simulink model "RADTRANS003"  (R2020b)
settings: Solver=VariableStepAuto  StartTime=0.0  StopTime=10.0  RelTol=1e-3
undefined symbols (not defined in the file): L_street, Line_110_C, Line_110_L, Line_110_R, Line_220_C, Line_220_L, Line_220_R, Line_35_C, Line_35_L, Line_35_R, Line_6_L, Line_6_R, P_nom_dyn, Q_nom_dyn, R_street, Sys_f_Hz, Sys_V_net_kV, Tr_110_35_L_pu, Tr_110_35_R_pu, Tr_110_35_Sn_VA, Tr_110_35_V_HV_kV, Tr_110_35_V_LV_kV, Tr_110_6_L_pu, Tr_110_6_R_pu, Tr_110_6_Sn_VA, Tr_110_6_V_HV_kV, Tr_110_6_V_LV_kV, Tr_220_110_L_pu, Tr_220_110_R_pu, Tr_220_110_Sn_VA, Tr_220_110_V_HV_kV, Tr_220_110_V_LV_kV, Tr_35_04_L_pu, Tr_35_04_R_pu, Tr_35_04_Sn_VA, Tr_35_04_V_HV_kV, Tr_35_04_V_LV_kV, Tr_6_04_L_pu, Tr_6_04_R_pu, Tr_6_04_Sn_VA, Tr_6_04_V_HV_kV, Tr_6_04_V_LV_kV, Ts_powergui
libraries: dspstat3 x96, powerlib x81, powerlib_meascontrol x24, simulink x2
(part 3 of 3)

== system RADTRANS003/M_OUT_Город_2_2 ==
  Iptg_20 : Display
      settings: Format=bank
  PQptg_20 : Scope  NumInputPorts=2
  "Power0 (3ph, Instantaneous)" : powerlib_meascontrol/Measurements/Power (3ph, Instantaneous)
  Pptg_20 : Display
      settings: Format=bank
  Qptg_20 : Display
      settings: Format=bank
  RMS20 : dspstat3/RMS  run=off  directionMode=Each column  dimension=1  InputProcessing=Columns as channels (frame based)  reset_popup=None
  RMS3 : dspstat3/RMS  run=off  directionMode=Each column  dimension=1  InputProcessing=Columns as channels (frame based)  reset_popup=None
  RMS4 : dspstat3/RMS  run=off  directionMode=Each column  dimension=1  InputProcessing=Columns as channels (frame based)  reset_popup=None
  RMSpt_20 : dspstat3/RMS  run=off  directionMode=Each column  dimension=1  InputProcessing=Columns as channels (frame based)  reset_popup=None
  Real-Ima to Complex : RealImagToComplex
  S : Abs
  SSptg_20 : Scope
  Sptg_20 : Display
      settings: Format=bank
  Three-Phase V-I Measurementpt_20 : powerlib/Measurements/Three-Phase V-I Measurement  VoltageMeasurement=phase-to-ground  SetLabelV=off  LabelV=Vabc  Vpu=off  VpuLL=off  CurrentMeasurement=yes  SetLabelI=off  LabelI=Iabc  Ipu=off  Pbase=100e6  Vbase=500e3  OutputType=Complex  PhasorSimulation=off  PSBequivalent=0
  UIptg_20 : Scope  NumInputPorts=2
  Uptg_20 : Display
      settings: Format=bank
  a : PMIOPort  Side=Right
  b : PMIOPort  Port=2  Side=Right
  c : PMIOPort  Port=3  Side=Right
  A : PMIOPort  Port=4  Side=Left
  B : PMIOPort  Port=5  Side=Left
  C : PMIOPort  Port=6  Side=Left
  tag scope: I_ptg_20=global, P_ptg_20=global, Q_ptg_20=global, S_ptg_20=global, U_ptg_20=global
  wires:
  S/1 -> [S_ptg_20]
  Real-Ima to Complex/1 -> S/1
  [S_ptg_20] -> Sptg_20/1
  [S_ptg_20] -> SSptg_20/1
  [P_ptg_20] -> RMSpt_20/1
  RMSpt_20/1 -> Pptg_20/1
  RMS20/1 -> Qptg_20/1
  [U_ptg_20] -> RMS3/1
  RMS3/1 -> Uptg_20/1
  [P_ptg_20] -> Real-Ima to Complex/1
  [Q_ptg_20] -> RMS20/1
  [I_ptg_20] -> RMS4/1
  RMS4/1 -> Iptg_20/1
  [U_ptg_20] -> UIptg_20/1  "U"
  [P_ptg_20] -> PQptg_20/1  "P"
  [I_ptg_20] -> UIptg_20/2  "I"
  Three-Phase V-I Measurementpt_20/1 -> [U_ptg_20]
  [Q_ptg_20] -> Real-Ima to Complex/2
  Three-Phase V-I Measurementpt_20/2 -> [I_ptg_20]
  [U_ptg_20] -> "Power0 (3ph, Instantaneous)"/1
  [I_ptg_20] -> "Power0 (3ph, Instantaneous)"/2
  "Power0 (3ph, Instantaneous)"/2 -> [Q_ptg_20]
  "Power0 (3ph, Instantaneous)"/1 -> [P_ptg_20]
  [Q_ptg_20] -> PQptg_20/2  "Q"
  connections:
  Three-Phase V-I Measurementpt_20/LConn1 -- A/RConn1
  Three-Phase V-I Measurementpt_20/RConn1 -- a/RConn1
  Three-Phase V-I Measurementpt_20/LConn2 -- B/RConn1
  Three-Phase V-I Measurementpt_20/LConn3 -- C/RConn1
  Three-Phase V-I Measurementpt_20/RConn3 -- c/RConn1
  Three-Phase V-I Measurementpt_20/RConn2 -- b/RConn1

== system RADTRANS003/M_OUT_Город_2_3 ==
  Iptg_22 : Display
      settings: Format=bank
  PQptg_22 : Scope  NumInputPorts=2
  "Power0 (3ph, Instantaneous)" : powerlib_meascontrol/Measurements/Power (3ph, Instantaneous)
  Pptg_22 : Display
      settings: Format=bank
  Qptg_22 : Display
      settings: Format=bank
  RMS22 : dspstat3/RMS  run=off  directionMode=Each column  dimension=1  InputProcessing=Columns as channels (frame based)  reset_popup=None
  RMS3 : dspstat3/RMS  run=off  directionMode=Each column  dimension=1  InputProcessing=Columns as channels (frame based)  reset_popup=None
  RMS4 : dspstat3/RMS  run=off  directionMode=Each column  dimension=1  InputProcessing=Columns as channels (frame based)  reset_popup=None
  RMSpt_22 : dspstat3/RMS  run=off  directionMode=Each column  dimension=1  InputProcessing=Columns as channels (frame based)  reset_popup=None
  Real-Ima to Complex : RealImagToComplex
  S : Abs
  SSptg_22 : Scope
  Sptg_22 : Display
      settings: Format=bank
  Three-Phase V-I Measurementpt_22 : powerlib/Measurements/Three-Phase V-I Measurement  VoltageMeasurement=phase-to-ground  SetLabelV=off  LabelV=Vabc  Vpu=off  VpuLL=off  CurrentMeasurement=yes  SetLabelI=off  LabelI=Iabc  Ipu=off  Pbase=100e6  Vbase=500e3  OutputType=Complex  PhasorSimulation=off  PSBequivalent=0
  UIptg_22 : Scope  NumInputPorts=2
  Uptg_22 : Display
      settings: Format=bank
  a : PMIOPort  Side=Right
  b : PMIOPort  Port=2  Side=Right
  c : PMIOPort  Port=3  Side=Right
  A : PMIOPort  Port=4  Side=Left
  B : PMIOPort  Port=5  Side=Left
  C : PMIOPort  Port=6  Side=Left
  tag scope: I_ptg_22=global, P_ptg_22=global, Q_ptg_22=global, S_ptg_22=global, U_ptg_22=global
  wires:
  S/1 -> [S_ptg_22]
  Real-Ima to Complex/1 -> S/1
  [S_ptg_22] -> Sptg_22/1
  [S_ptg_22] -> SSptg_22/1
  [P_ptg_22] -> RMSpt_22/1
  RMSpt_22/1 -> Pptg_22/1
  RMS22/1 -> Qptg_22/1
  [U_ptg_22] -> RMS3/1
  RMS3/1 -> Uptg_22/1
  [P_ptg_22] -> Real-Ima to Complex/1
  [Q_ptg_22] -> RMS22/1
  [I_ptg_22] -> RMS4/1
  RMS4/1 -> Iptg_22/1
  [U_ptg_22] -> UIptg_22/1  "U"
  [P_ptg_22] -> PQptg_22/1  "P"
  [I_ptg_22] -> UIptg_22/2  "I"
  Three-Phase V-I Measurementpt_22/1 -> [U_ptg_22]
  [Q_ptg_22] -> Real-Ima to Complex/2
  Three-Phase V-I Measurementpt_22/2 -> [I_ptg_22]
  [U_ptg_22] -> "Power0 (3ph, Instantaneous)"/1
  [I_ptg_22] -> "Power0 (3ph, Instantaneous)"/2
  "Power0 (3ph, Instantaneous)"/2 -> [Q_ptg_22]
  "Power0 (3ph, Instantaneous)"/1 -> [P_ptg_22]
  [Q_ptg_22] -> PQptg_22/2  "Q"
  connections:
  Three-Phase V-I Measurementpt_22/LConn1 -- A/RConn1
  Three-Phase V-I Measurementpt_22/RConn1 -- a/RConn1
  Three-Phase V-I Measurementpt_22/LConn2 -- B/RConn1
  Three-Phase V-I Measurementpt_22/LConn3 -- C/RConn1
  Three-Phase V-I Measurementpt_22/RConn3 -- c/RConn1
  Three-Phase V-I Measurementpt_22/RConn2 -- b/RConn1

== system RADTRANS003/M_OUT_Город_2_4 ==
  Iptg_24 : Display
      settings: Format=bank
  PQptg_24 : Scope  NumInputPorts=2
  "Power0 (3ph, Instantaneous)" : powerlib_meascontrol/Measurements/Power (3ph, Instantaneous)
  Pptg_24 : Display
      settings: Format=bank
  Qptg_24 : Display
      settings: Format=bank
  RMS24 : dspstat3/RMS  run=off  directionMode=Each column  dimension=1  InputProcessing=Columns as channels (frame based)  reset_popup=None
  RMS3 : dspstat3/RMS  run=off  directionMode=Each column  dimension=1  InputProcessing=Columns as channels (frame based)  reset_popup=None
  RMS4 : dspstat3/RMS  run=off  directionMode=Each column  dimension=1  InputProcessing=Columns as channels (frame based)  reset_popup=None
  RMSpt_24 : dspstat3/RMS  run=off  directionMode=Each column  dimension=1  InputProcessing=Columns as channels (frame based)  reset_popup=None
  Real-Ima to Complex : RealImagToComplex
  S : Abs
  SSptg_24 : Scope
  Sptg_24 : Display
      settings: Format=bank
  Three-Phase V-I Measurementpt_24 : powerlib/Measurements/Three-Phase V-I Measurement  VoltageMeasurement=phase-to-ground  SetLabelV=off  LabelV=Vabc  Vpu=off  VpuLL=off  CurrentMeasurement=yes  SetLabelI=off  LabelI=Iabc  Ipu=off  Pbase=100e6  Vbase=500e3  OutputType=Complex  PhasorSimulation=off  PSBequivalent=0
  UIptg_24 : Scope  NumInputPorts=2
  Uptg_24 : Display
      settings: Format=bank
  a : PMIOPort  Side=Right
  b : PMIOPort  Port=2  Side=Right
  c : PMIOPort  Port=3  Side=Right
  A : PMIOPort  Port=4  Side=Left
  B : PMIOPort  Port=5  Side=Left
  C : PMIOPort  Port=6  Side=Left
  tag scope: I_ptg_24=global, P_ptg_24=global, Q_ptg_24=global, S_ptg_24=global, U_ptg_24=global
  wires:
  S/1 -> [S_ptg_24]
  Real-Ima to Complex/1 -> S/1
  [S_ptg_24] -> Sptg_24/1
  [S_ptg_24] -> SSptg_24/1
  [P_ptg_24] -> RMSpt_24/1
  RMSpt_24/1 -> Pptg_24/1
  RMS24/1 -> Qptg_24/1
  [U_ptg_24] -> RMS3/1
  RMS3/1 -> Uptg_24/1
  [P_ptg_24] -> Real-Ima to Complex/1
  [Q_ptg_24] -> RMS24/1
  [I_ptg_24] -> RMS4/1
  RMS4/1 -> Iptg_24/1
  [U_ptg_24] -> UIptg_24/1  "U"
  [P_ptg_24] -> PQptg_24/1  "P"
  [I_ptg_24] -> UIptg_24/2  "I"
  Three-Phase V-I Measurementpt_24/1 -> [U_ptg_24]
  [Q_ptg_24] -> Real-Ima to Complex/2
  Three-Phase V-I Measurementpt_24/2 -> [I_ptg_24]
  [U_ptg_24] -> "Power0 (3ph, Instantaneous)"/1
  [I_ptg_24] -> "Power0 (3ph, Instantaneous)"/2
  "Power0 (3ph, Instantaneous)"/2 -> [Q_ptg_24]
  "Power0 (3ph, Instantaneous)"/1 -> [P_ptg_24]
  [Q_ptg_24] -> PQptg_24/2  "Q"
  connections:
  Three-Phase V-I Measurementpt_24/LConn1 -- A/RConn1
  Three-Phase V-I Measurementpt_24/RConn1 -- a/RConn1
  Three-Phase V-I Measurementpt_24/LConn2 -- B/RConn1
  Three-Phase V-I Measurementpt_24/LConn3 -- C/RConn1
  Three-Phase V-I Measurementpt_24/RConn3 -- c/RConn1
  Three-Phase V-I Measurementpt_24/RConn2 -- b/RConn1

== system RADTRANS003/M_OUT_Завод_1_1 ==
  Iptg_2 : Display
      settings: Format=bank
  PQptg_2 : Scope  NumInputPorts=2
  "Power0 (3ph, Instantaneous)" : powerlib_meascontrol/Measurements/Power (3ph, Instantaneous)
  Pptg_2 : Display
      settings: Format=bank
  Qptg_2 : Display
      settings: Format=bank
  RMS2 : dspstat3/RMS  run=off  directionMode=Each column  dimension=1  InputProcessing=Columns as channels (frame based)  reset_popup=None
  RMS3 : dspstat3/RMS  run=off  directionMode=Each column  dimension=1  InputProcessing=Columns as channels (frame based)  reset_popup=None
  RMS4 : dspstat3/RMS  run=off  directionMode=Each column  dimension=1  InputProcessing=Columns as channels (frame based)  reset_popup=None
  RMSpt_2 : dspstat3/RMS  run=off  directionMode=Each column  dimension=1  InputProcessing=Columns as channels (frame based)  reset_popup=None
  Real-Ima to Complex : RealImagToComplex
  S : Abs
  SSptg_2 : Scope
  Sptg_2 : Display
      settings: Format=bank
  Three-Phase V-I Measurementpt_2 : powerlib/Measurements/Three-Phase V-I Measurement  VoltageMeasurement=phase-to-ground  SetLabelV=off  LabelV=Vabc  Vpu=off  VpuLL=off  CurrentMeasurement=yes  SetLabelI=off  LabelI=Iabc  Ipu=off  Pbase=100e6  Vbase=500e3  OutputType=Complex  PhasorSimulation=off  PSBequivalent=0
  UIptg_2 : Scope  NumInputPorts=2
  Uptg_2 : Display
      settings: Format=bank
  a : PMIOPort  Side=Right
  b : PMIOPort  Port=2  Side=Right
  c : PMIOPort  Port=3  Side=Right
  A : PMIOPort  Port=4  Side=Left
  B : PMIOPort  Port=5  Side=Left
  C : PMIOPort  Port=6  Side=Left
  tag scope: I_ptg_2=global, P_ptg_2=global, Q_ptg_2=global, S_ptg_2=global, U_ptg_2=global
  wires:
  S/1 -> [S_ptg_2]
  Real-Ima to Complex/1 -> S/1
  [S_ptg_2] -> Sptg_2/1
  [S_ptg_2] -> SSptg_2/1
  [P_ptg_2] -> RMSpt_2/1
  RMSpt_2/1 -> Pptg_2/1
  RMS2/1 -> Qptg_2/1
  [U_ptg_2] -> RMS3/1
  RMS3/1 -> Uptg_2/1
  [P_ptg_2] -> Real-Ima to Complex/1
  [Q_ptg_2] -> RMS2/1
  [I_ptg_2] -> RMS4/1
  RMS4/1 -> Iptg_2/1
  [U_ptg_2] -> UIptg_2/1  "U"
  [P_ptg_2] -> PQptg_2/1  "P"
  [I_ptg_2] -> UIptg_2/2  "I"
  Three-Phase V-I Measurementpt_2/1 -> [U_ptg_2]
  [Q_ptg_2] -> Real-Ima to Complex/2
  Three-Phase V-I Measurementpt_2/2 -> [I_ptg_2]
  [U_ptg_2] -> "Power0 (3ph, Instantaneous)"/1
  [I_ptg_2] -> "Power0 (3ph, Instantaneous)"/2
  "Power0 (3ph, Instantaneous)"/2 -> [Q_ptg_2]
  "Power0 (3ph, Instantaneous)"/1 -> [P_ptg_2]
  [Q_ptg_2] -> PQptg_2/2  "Q"
  connections:
  Three-Phase V-I Measurementpt_2/LConn1 -- A/RConn1
  Three-Phase V-I Measurementpt_2/RConn1 -- a/RConn1
  Three-Phase V-I Measurementpt_2/LConn2 -- B/RConn1
  Three-Phase V-I Measurementpt_2/LConn3 -- C/RConn1
  Three-Phase V-I Measurementpt_2/RConn3 -- c/RConn1
  Three-Phase V-I Measurementpt_2/RConn2 -- b/RConn1

== system RADTRANS003/M_OUT_Завод_1_2 ==
  Iptg_4 : Display
      settings: Format=bank
  PQptg_4 : Scope  NumInputPorts=2
  "Power0 (3ph, Instantaneous)" : powerlib_meascontrol/Measurements/Power (3ph, Instantaneous)
  Pptg_4 : Display
      settings: Format=bank
  Qptg_4 : Display
      settings: Format=bank
  RMS0 : dspstat3/RMS  run=off  directionMode=Each column  dimension=1  InputProcessing=Columns as channels (frame based)  reset_popup=None
  RMS3 : dspstat3/RMS  run=off  directionMode=Each column  dimension=1  InputProcessing=Columns as channels (frame based)  reset_popup=None
  RMS4 : dspstat3/RMS  run=off  directionMode=Each column  dimension=1  InputProcessing=Columns as channels (frame based)  reset_popup=None
  RMSpt_4 : dspstat3/RMS  run=off  directionMode=Each column  dimension=1  InputProcessing=Columns as channels (frame based)  reset_popup=None
  Real-Ima to Complex : RealImagToComplex
  S : Abs
  SSptg_4 : Scope
  Sptg_4 : Display
      settings: Format=bank
  Three-Phase V-I Measurementpt_4 : powerlib/Measurements/Three-Phase V-I Measurement  VoltageMeasurement=phase-to-ground  SetLabelV=off  LabelV=Vabc  Vpu=off  VpuLL=off  CurrentMeasurement=yes  SetLabelI=off  LabelI=Iabc  Ipu=off  Pbase=100e6  Vbase=500e3  OutputType=Complex  PhasorSimulation=off  PSBequivalent=0
  UIptg_4 : Scope  NumInputPorts=2
  Uptg_4 : Display
      settings: Format=bank
  a : PMIOPort  Side=Right
  b : PMIOPort  Port=2  Side=Right
  c : PMIOPort  Port=3  Side=Right
  A : PMIOPort  Port=4  Side=Left
  B : PMIOPort  Port=5  Side=Left
  C : PMIOPort  Port=6  Side=Left
  tag scope: I_ptg_4=global, P_ptg_4=global, Q_ptg_4=global, S_ptg_4=global, U_ptg_4=global
  wires:
  S/1 -> [S_ptg_4]
  Real-Ima to Complex/1 -> S/1
  [S_ptg_4] -> Sptg_4/1
  [S_ptg_4] -> SSptg_4/1
  [P_ptg_4] -> RMSpt_4/1
  RMSpt_4/1 -> Pptg_4/1
  RMS0/1 -> Qptg_4/1
  [U_ptg_4] -> RMS3/1
  RMS3/1 -> Uptg_4/1
  [P_ptg_4] -> Real-Ima to Complex/1
  [Q_ptg_4] -> RMS0/1
  [I_ptg_4] -> RMS4/1
  RMS4/1 -> Iptg_4/1
  [U_ptg_4] -> UIptg_4/1  "U"
  [P_ptg_4] -> PQptg_4/1  "P"
  [I_ptg_4] -> UIptg_4/2  "I"
  Three-Phase V-I Measurementpt_4/1 -> [U_ptg_4]
  [Q_ptg_4] -> Real-Ima to Complex/2
  Three-Phase V-I Measurementpt_4/2 -> [I_ptg_4]
  [U_ptg_4] -> "Power0 (3ph, Instantaneous)"/1
  [I_ptg_4] -> "Power0 (3ph, Instantaneous)"/2
  "Power0 (3ph, Instantaneous)"/2 -> [Q_ptg_4]
  "Power0 (3ph, Instantaneous)"/1 -> [P_ptg_4]
  [Q_ptg_4] -> PQptg_4/2  "Q"
  connections:
  Three-Phase V-I Measurementpt_4/LConn1 -- A/RConn1
  Three-Phase V-I Measurementpt_4/RConn1 -- a/RConn1
  Three-Phase V-I Measurementpt_4/LConn2 -- B/RConn1
  Three-Phase V-I Measurementpt_4/LConn3 -- C/RConn1
  Three-Phase V-I Measurementpt_4/RConn3 -- c/RConn1
  Three-Phase V-I Measurementpt_4/RConn2 -- b/RConn1

== system RADTRANS003/M_OUT_Завод_2_1 ==
  Iptg_14 : Display
      settings: Format=bank
  PQptg_14 : Scope  NumInputPorts=2
  "Power0 (3ph, Instantaneous)" : powerlib_meascontrol/Measurements/Power (3ph, Instantaneous)
  Pptg_14 : Display
      settings: Format=bank
  Qptg_14 : Display
      settings: Format=bank
  RMS14 : dspstat3/RMS  run=off  directionMode=Each column  dimension=1  InputProcessing=Columns as channels (frame based)  reset_popup=None
  RMS3 : dspstat3/RMS  run=off  directionMode=Each column  dimension=1  InputProcessing=Columns as channels (frame based)  reset_popup=None
  RMS4 : dspstat3/RMS  run=off  directionMode=Each column  dimension=1  InputProcessing=Columns as channels (frame based)  reset_popup=None
  RMSpt_14 : dspstat3/RMS  run=off  directionMode=Each column  dimension=1  InputProcessing=Columns as channels (frame based)  reset_popup=None
  Real-Ima to Complex : RealImagToComplex
  S : Abs
  SSptg_14 : Scope
  Sptg_14 : Display
      settings: Format=bank
  Three-Phase V-I Measurementpt_14 : powerlib/Measurements/Three-Phase V-I Measurement  VoltageMeasurement=phase-to-ground  SetLabelV=off  LabelV=Vabc  Vpu=off  VpuLL=off  CurrentMeasurement=yes  SetLabelI=off  LabelI=Iabc  Ipu=off  Pbase=100e6  Vbase=500e3  OutputType=Complex  PhasorSimulation=off  PSBequivalent=0
  UIptg_14 : Scope  NumInputPorts=2
  Uptg_14 : Display
      settings: Format=bank
  a : PMIOPort  Side=Right
  b : PMIOPort  Port=2  Side=Right
  c : PMIOPort  Port=3  Side=Right
  A : PMIOPort  Port=4  Side=Left
  B : PMIOPort  Port=5  Side=Left
  C : PMIOPort  Port=6  Side=Left
  tag scope: I_ptg_14=global, P_ptg_14=global, Q_ptg_14=global, S_ptg_14=global, U_ptg_14=global
  wires:
  S/1 -> [S_ptg_14]
  Real-Ima to Complex/1 -> S/1
  [S_ptg_14] -> Sptg_14/1
  [S_ptg_14] -> SSptg_14/1
  [P_ptg_14] -> RMSpt_14/1
  RMSpt_14/1 -> Pptg_14/1
  RMS14/1 -> Qptg_14/1
  [U_ptg_14] -> RMS3/1
  RMS3/1 -> Uptg_14/1
  [P_ptg_14] -> Real-Ima to Complex/1
  [Q_ptg_14] -> RMS14/1
  [I_ptg_14] -> RMS4/1
  RMS4/1 -> Iptg_14/1
  [U_ptg_14] -> UIptg_14/1  "U"
  [P_ptg_14] -> PQptg_14/1  "P"
  [I_ptg_14] -> UIptg_14/2  "I"
  Three-Phase V-I Measurementpt_14/1 -> [U_ptg_14]
  [Q_ptg_14] -> Real-Ima to Complex/2
  Three-Phase V-I Measurementpt_14/2 -> [I_ptg_14]
  [U_ptg_14] -> "Power0 (3ph, Instantaneous)"/1
  [I_ptg_14] -> "Power0 (3ph, Instantaneous)"/2
  "Power0 (3ph, Instantaneous)"/2 -> [Q_ptg_14]
  "Power0 (3ph, Instantaneous)"/1 -> [P_ptg_14]
  [Q_ptg_14] -> PQptg_14/2  "Q"
  connections:
  Three-Phase V-I Measurementpt_14/LConn1 -- A/RConn1
  Three-Phase V-I Measurementpt_14/RConn1 -- a/RConn1
  Three-Phase V-I Measurementpt_14/LConn2 -- B/RConn1
  Three-Phase V-I Measurementpt_14/LConn3 -- C/RConn1
  Three-Phase V-I Measurementpt_14/RConn3 -- c/RConn1
  Three-Phase V-I Measurementpt_14/RConn2 -- b/RConn1

== system RADTRANS003/M_OUT_Завод_2_2 ==
  Iptg_16 : Display
      settings: Format=bank
  PQptg_16 : Scope  NumInputPorts=2
  "Power0 (3ph, Instantaneous)" : powerlib_meascontrol/Measurements/Power (3ph, Instantaneous)
  Pptg_16 : Display
      settings: Format=bank
  Qptg_16 : Display
      settings: Format=bank
  RMS16 : dspstat3/RMS  run=off  directionMode=Each column  dimension=1  InputProcessing=Columns as channels (frame based)  reset_popup=None
  RMS3 : dspstat3/RMS  run=off  directionMode=Each column  dimension=1  InputProcessing=Columns as channels (frame based)  reset_popup=None
  RMS4 : dspstat3/RMS  run=off  directionMode=Each column  dimension=1  InputProcessing=Columns as channels (frame based)  reset_popup=None
  RMSpt_16 : dspstat3/RMS  run=off  directionMode=Each column  dimension=1  InputProcessing=Columns as channels (frame based)  reset_popup=None
  Real-Ima to Complex : RealImagToComplex
  S : Abs
  SSptg_16 : Scope
  Sptg_16 : Display
      settings: Format=bank
  Three-Phase V-I Measurementpt_16 : powerlib/Measurements/Three-Phase V-I Measurement  VoltageMeasurement=phase-to-ground  SetLabelV=off  LabelV=Vabc  Vpu=off  VpuLL=off  CurrentMeasurement=yes  SetLabelI=off  LabelI=Iabc  Ipu=off  Pbase=100e6  Vbase=500e3  OutputType=Complex  PhasorSimulation=off  PSBequivalent=0
  UIptg_16 : Scope  NumInputPorts=2
  Uptg_16 : Display
      settings: Format=bank
  a : PMIOPort  Side=Right
  b : PMIOPort  Port=2  Side=Right
  c : PMIOPort  Port=3  Side=Right
  A : PMIOPort  Port=4  Side=Left
  B : PMIOPort  Port=5  Side=Left
  C : PMIOPort  Port=6  Side=Left
  tag scope: I_ptg_16=global, P_ptg_16=global, Q_ptg_16=global, S_ptg_16=global, U_ptg_16=global
  wires:
  S/1 -> [S_ptg_16]
  Real-Ima to Complex/1 -> S/1
  [S_ptg_16] -> Sptg_16/1
  [S_ptg_16] -> SSptg_16/1
  [P_ptg_16] -> RMSpt_16/1
  RMSpt_16/1 -> Pptg_16/1
  RMS16/1 -> Qptg_16/1
  [U_ptg_16] -> RMS3/1
  RMS3/1 -> Uptg_16/1
  [P_ptg_16] -> Real-Ima to Complex/1
  [Q_ptg_16] -> RMS16/1
  [I_ptg_16] -> RMS4/1
  RMS4/1 -> Iptg_16/1
  [U_ptg_16] -> UIptg_16/1  "U"
  [P_ptg_16] -> PQptg_16/1  "P"
  [I_ptg_16] -> UIptg_16/2  "I"
  Three-Phase V-I Measurementpt_16/1 -> [U_ptg_16]
  [Q_ptg_16] -> Real-Ima to Complex/2
  Three-Phase V-I Measurementpt_16/2 -> [I_ptg_16]
  [U_ptg_16] -> "Power0 (3ph, Instantaneous)"/1
  [I_ptg_16] -> "Power0 (3ph, Instantaneous)"/2
  "Power0 (3ph, Instantaneous)"/2 -> [Q_ptg_16]
  "Power0 (3ph, Instantaneous)"/1 -> [P_ptg_16]
  [Q_ptg_16] -> PQptg_16/2  "Q"
  connections:
  Three-Phase V-I Measurementpt_16/LConn1 -- A/RConn1
  Three-Phase V-I Measurementpt_16/RConn1 -- a/RConn1
  Three-Phase V-I Measurementpt_16/LConn2 -- B/RConn1
  Three-Phase V-I Measurementpt_16/LConn3 -- C/RConn1
  Three-Phase V-I Measurementpt_16/RConn3 -- c/RConn1
  Three-Phase V-I Measurementpt_16/RConn2 -- b/RConn1
